simulink model "EDR_Unit"  (R2020b)
settings: configuration reference "unit_config" (kept outside this file)
libraries: simulink_extras x1
settings Model: DataDictionary=Hybrid_vehicle_update.sldd  SimulationMode=accelerator  Creator=Georg  LastModifiedBy=jy
settings ConfigSetRef: SourceName=unit_config

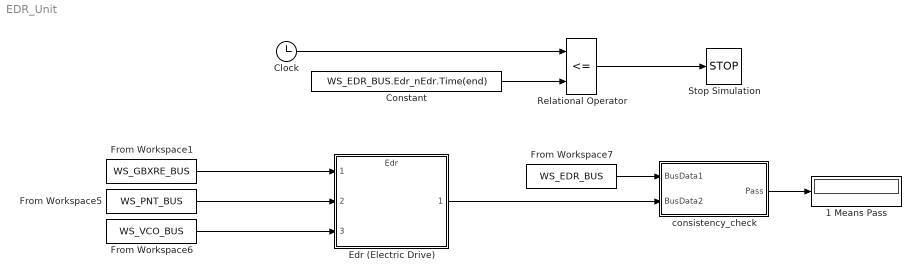
== system EDR_Unit ==
  1 Means Pass : Display
  Clock : Clock
  Constant : Constant  Value=WS_EDR_BUS.Edr_nEdr.Time(end)
  Edr (Electric Drive) : ModelReference  ModelNameDialog=Edr  SimulationMode=Normal  ModelReferenceVersion=2.16
      mask Display: image('$imagefile'); % Use "Edit Image" on toolstrip to change.
  From Workspace1 : FromWorkspace  VariableName=WS_GBXRE_BUS  OutDataTypeStr=Bus: GBXRE_BUS  SampleTime=0.002  Interpolate=off  OutputAfterFinalValue=Holding final value
  From Workspace5 : FromWorkspace  VariableName=WS_PNT_BUS  OutDataTypeStr=Bus: PNT_BUS  SampleTime=0.002  Interpolate=off  OutputAfterFinalValue=Holding final value
  From Workspace6 : FromWorkspace  VariableName=WS_VCO_BUS  OutDataTypeStr=Bus: VCO_BUS  SampleTime=0.002  Interpolate=off  OutputAfterFinalValue=Holding final value
  From Workspace7 : FromWorkspace  VariableName=WS_EDR_BUS  OutDataTypeStr=Bus: EDR_BUS  SampleTime=0.002  Interpolate=off  OutputAfterFinalValue=Holding final value
  Relational Operator : RelationalOperator  Operator=<=  OutDataTypeStr=boolean  RndMeth=Simplest
  Stop Simulation : Stop
  consistency_check : Subsystem
  wires:
  Clock/1 -> Relational Operator/1
  Relational Operator/1 -> Stop Simulation/1
  Constant/1 -> Relational Operator/2
  From Workspace1/1 -> Edr (Electric Drive)/1
  From Workspace5/1 -> Edr (Electric Drive)/2
  From Workspace6/1 -> Edr (Electric Drive)/3
  Edr (Electric Drive)/1 -> consistency_check/2(BusData2)
  From Workspace7/1 -> consistency_check/1(BusData1)
  consistency_check/1(Pass) -> 1 Means Pass/1

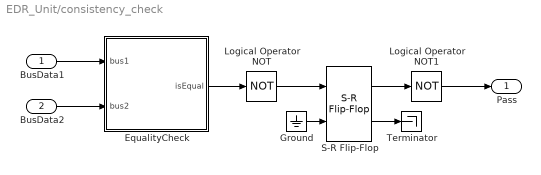
== system EDR_Unit/consistency_check ==
  BusData1 : Inport
  BusData2 : Inport  Port=2
  EqualityCheck : MATLAB Function  TreatAsAtomicUnit=on
  Ground : Ground
  Logical Operator NOT : Logic  Operator=NOT  AllPortsSameDT=off  OutDataTypeStr=boolean
  Logical Operator NOT1 : Logic  Operator=NOT  AllPortsSameDT=off  OutDataTypeStr=boolean
  S-R Flip-Flop : simulink_extras/Flip Flops/S-R Flip-Flop  initial_condition=0
  Terminator : Terminator
  Pass : Outport  VectorParamsAs1DForOutWhenUnconnected=off
  wires:
  Logical Operator NOT1/1 -> Pass/1
  S-R Flip-Flop/1 -> Logical Operator NOT1/1
  S-R Flip-Flop/2 -> Terminator/1
  Ground/1 -> S-R Flip-Flop/2
  Logical Operator NOT/1 -> S-R Flip-Flop/1
  EqualityCheck/1(isEqual) -> Logical Operator NOT/1
  BusData2/1 -> EqualityCheck/2(bus2)
  BusData1/1 -> EqualityCheck/1(bus1)

== matlab function EDR_Unit/consistency_check/EqualityCheck ==
  data: bus1 input; isEqual output; bus2 input
function isEqual = fcn(bus1, bus2)
isEqual = isequal(bus1, bus2);
